simulink model "regulator_LQG_1"  (R2021b)
settings: Solver=VariableStepAuto  StartTime=0.0  StopTime=10.0  RelTol=1e-3
values from neighbouring files (symbols this model uses):
  C_temp = eye(length(A))    [main2.m]
  D_temp = zeros(length(B), 1)    [main2.m]
  x0 = [0 10]    [main2.m]
undefined symbols (not defined in the file or in its folder): A, B, C, Continuous, k_LQ, Time
libraries: simulink x2, ctrlSharedLib x1
settings Model: Creator=PaoloA  LastModifiedBy=PaoloA

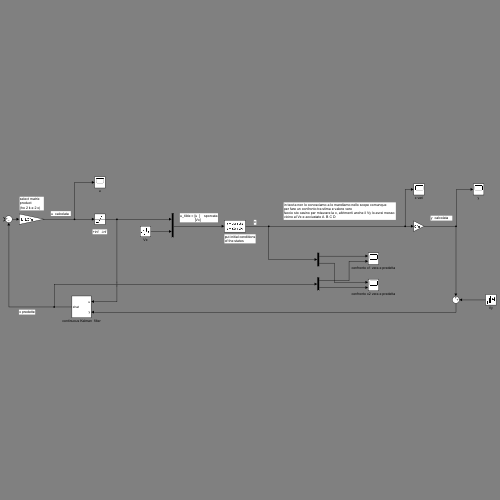
[thumbnail: Simulink's stored preview of the top-level diagram]
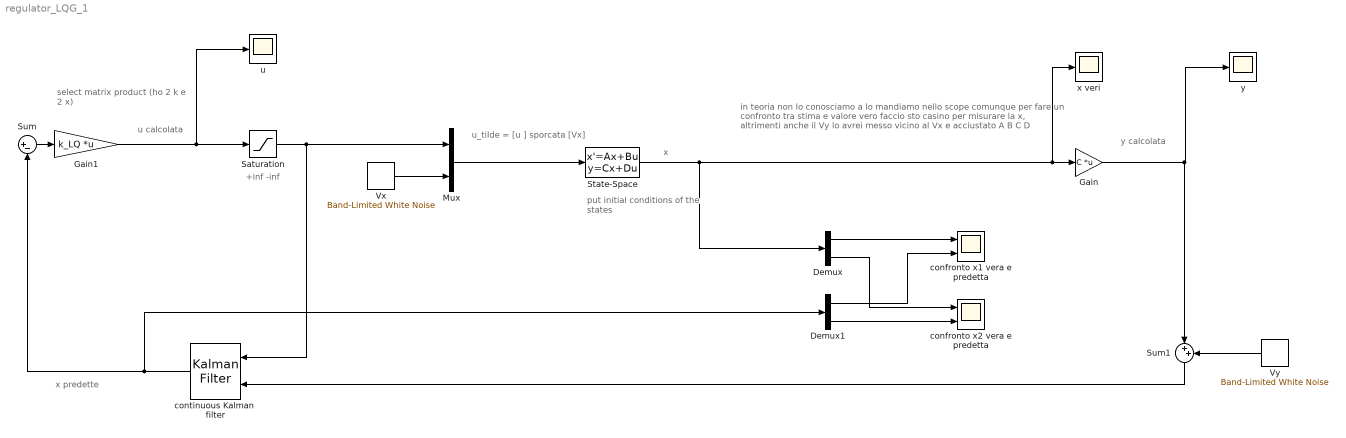
== system regulator_LQG_1 ==
  note: u_tilde = [u  ]    sporcata
      |                [Vx]
  note: x predette
  note: in teoria non lo conosciamo a lo mandiamo nello scope comunque
      | per fare un confronto tra stima e valore vero
      | faccio sto casino per misurare la x, altrimenti anche il Vy lo avrei messo
      | vicino al Vx e acciustato A  B C D
  note: select matrix
      | product
      | (ho 2 k e 2 x)
  note: y calcolata
  note: x
  note: u calcolata
  note: put initial conditions
      | of the states
  note: +inf -inf
  Demux : Demux  Outputs=2
  Demux1 : Demux  Outputs=2
  Gain : Gain  Gain=C  Multiplication=Matrix(K*u)
  Gain1 : Gain  Gain=k_LQ  Multiplication=Matrix(K*u)
  Mux : Mux  Inputs=2
  Saturation : Saturate  UpperLimit=+inf  LowerLimit=-inf
  State-Space : StateSpace  A=A  B=B  C=C_temp  D=D_temp  InitialCondition=x0
  Sum : Sum  Inputs=|+-
  Sum1 : Sum  Inputs=|++
  Vx : simulink/Sources/Band-Limited White Noise  Cov=[0.1]  Ts=0.1  seed=[23341]
  Vy : simulink/Sources/Band-Limited White Noise  Cov=[0.1]  Ts=0.1  seed=[23341]
  confronto x1 vera e predetta : Scope  NumInputPorts=2
  confronto x2 vera e predetta : Scope  NumInputPorts=2
  continuous Kalman  filter : ctrlSharedLib/Kalman Filter  TimeDomain=Continuous-Time  UseCurrentEstimator=on  ModelSource=Individual A, B, C, D matrices  ModelSourceVariable=ss(0.95,1,1,0,1)  A=0.95  B=1  C=1  D=0  NumberOfStates=1  NumberOfInputs=1  NumberOfOutputs=1  InitialEstimateSource=Dialog  X0=0  P0=10  UseK=off  UseGH=off  NumberOfProcessNoiseInputs=1  G=1  TimeInvariantG=on  H=0  TimeInvariantH=on  Q=0.05  TimeInvariantQ=on  R=1  TimeInvariantR=on  N=0  TimeInvariantN=on  AddInputPort=on  AddEnablePort=off  OutputEstimatedY=off  OutputP=off  Ts=-1
  u : Scope
  x veri : Scope
  y : Scope
  wires:
  Gain/1 -> y/1, Sum1/1
  Sum/1 -> Gain1/1
  Gain1/1 -> u/1, Saturation/1
  Saturation/1 -> continuous Kalman  filter/1, Mux/1
  State-Space/1 -> Demux/1, Gain/1, x veri/1
  continuous Kalman  filter/1 -> Demux1/1, Sum/2
  Sum1/1 -> continuous Kalman  filter/2
  Vx/1 -> Mux/2
  Mux/1 -> State-Space/1
  Demux/1 -> confronto x1 vera e predetta/1
  Demux1/1 -> confronto x1 vera e predetta/2
  Demux/2 -> confronto x2 vera e predetta/1
  Demux1/2 -> confronto x2 vera e predetta/2
  Vy/1 -> Sum1/2
